simulink model "quartercar_model"  (R2023a)
settings: Solver=VariableStepAuto  StartTime=0.0  StopTime=10.0  RelTol=1e-3
settings Model: Creator=NGOC MAI  LastModifiedBy=NGOC MAI

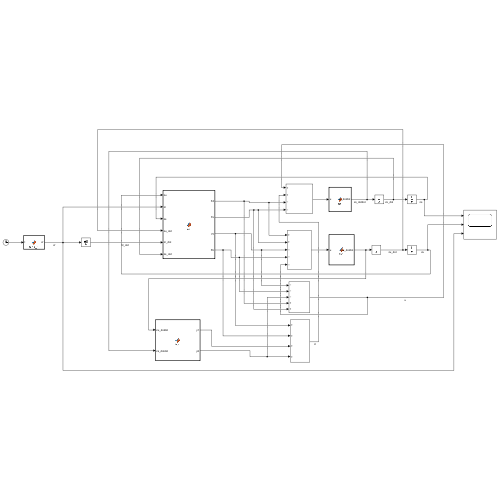
[thumbnail: Simulink's stored preview of the top-level diagram]
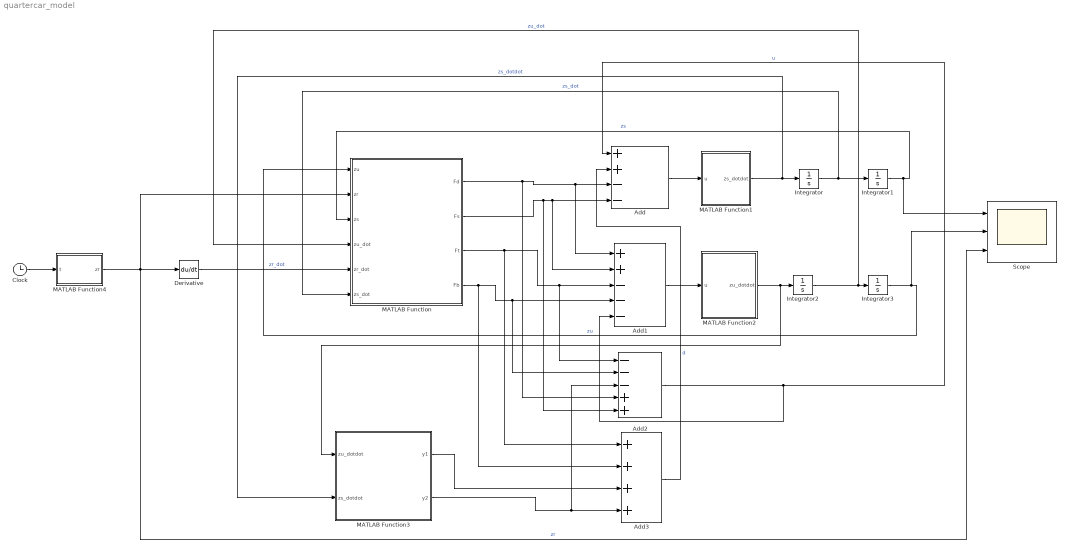
== system quartercar_model ==
  Add : Sum  Inputs=++--
  Add1 : Sum  Inputs=++---
  Add2 : Sum  Inputs=---++
  Add3 : Sum  Inputs=++++
  Clock : Clock
  Derivative : Derivative
  Integrator : Integrator
  Integrator1 : Integrator  InitialCondition=0.03
  Integrator2 : Integrator
  Integrator3 : Integrator
  MATLAB Function : MATLAB Function  TreatAsAtomicUnit=on
  MATLAB Function1 : MATLAB Function  TreatAsAtomicUnit=on
  MATLAB Function2 : MATLAB Function  TreatAsAtomicUnit=on
  MATLAB Function3 : MATLAB Function  TreatAsAtomicUnit=on
  MATLAB Function4 : MATLAB Function  TreatAsAtomicUnit=on
  Scope : Scope  NumInputPorts=3
  wires:
  MATLAB Function/1(Fd) -> Add2/4, Add1/1, Add/3
  Add/1 -> MATLAB Function1/1(u)
  MATLAB Function1/1(zs_dotdot) -> MATLAB Function3/2(zs_dotdot), Integrator/1  "zs_dotdot"
  Integrator/1 -> MATLAB Function/6(zs_dot), Integrator1/1  "zs_dot"
  Integrator1/1 -> Scope/1, MATLAB Function/3(zs)  "zs"
  Add2/1 -> Add/1, Add1/5  "u"
  Add3/1 -> Add/2  "d"
  MATLAB Function2/1(zu_dotdot) -> MATLAB Function3/1(zu_dotdot), Integrator2/1
  Integrator2/1 -> MATLAB Function/4(zu_dot), Integrator3/1  "zu_dot"
  Integrator3/1 -> Scope/2, MATLAB Function/1(zu)  "zu"
  MATLAB Function/2(Fs) -> Add2/5, Add1/2, Add/4
  MATLAB Function/3(Ft) -> Add3/1, Add2/1, Add1/3
  MATLAB Function/4(Fb) -> Add3/2, Add1/4, Add2/2
  Add1/1 -> MATLAB Function2/1(u)
  MATLAB Function3/1(y1) -> Add3/3
  MATLAB Function3/2(y2) -> Add2/3, Add3/4
  MATLAB Function4/1(zr) -> Scope/3, MATLAB Function/2(zr), Derivative/1  "zr"
  Derivative/1 -> MATLAB Function/5(zr_dot)  "zr_dot"
  Clock/1 -> MATLAB Function4/1(t)

== matlab function quartercar_model/MATLAB Function1 ==
  data: u input; zs_dotdot output
function zs_dotdot = fcn(u)
ms=600; %kg
zs_dotdot=u*(1/ms);
end

== matlab function quartercar_model/MATLAB Function ==
  data: zu input; zr input; zs input; zu_dot input; zr_dot input; zs_dot input; Fd output; Fs output; Ft output; Fb output
function [Fd,Fs,Ft,Fb]=fcn(zu,zr,zs,zu_dot,zr_dot,zs_dot)
ks=18000; %N/m
ksn=1000; %N/m
bc=2500; %Ns/m
kf=200000; %N/m
cf=1000; %Ns/m

delta_z = zs-zu; 

delta_zdot =  zs_dot-zu_dot;

Fs = ks*delta_z+ksn*delta_z^3;

Fd = bc*delta_zdot;

Ft = kf*(zu-zr);

Fb = cf*(zu_dot-zr_dot);

end

== matlab function quartercar_model/MATLAB Function2 ==
  data: u input; zu_dotdot output
function zu_dotdot = fcn(u)
mu=60; %kg
zu_dotdot=u*(1/mu);
end

== matlab function quartercar_model/MATLAB Function3 ==
  data: zu_dotdot input; y1 output; zs_dotdot input; y2 output
function [y1,y2] = fcn(zu_dotdot,zs_dotdot)
ms=600; %kg
mu=60; %kg
y1=ms*zs_dotdot;
y2=mu*zu_dotdot;
end

== matlab function quartercar_model/MATLAB Function4 ==
  data: t input; zr output
function zr = func_1(t)
   if t< 3.0
       zr = 0.0;
   elseif t< 3.5
       zr = 0.04*(1-cos(4*pi*t));
   else
       zr = 0;
   end
end
